simulink model "velocityform"  (R2024a)
settings: Solver=VariableStepAuto  StartTime=0.0  StopTime=10.0  RelTol=1e-3
values from neighbouring files (symbols this model uses):
  B_noise_real = [Bd ones(size(Bd,1),1)]    [scriptpoint7.m]
  D_noise_real = [Dd zeros(size(Dd,1),1)]    [scriptpoint7.m]
  N = 5    [project_script.m]    (also in scriptpoint7.m)
  NK = 0    [scriptpoint7.m]
  Qd = 1*eye(2)    [project_script.m]    (also in scriptpoint7.m = 1000*eye(2))
  Rd = 1*eye(2)    [project_script.m]    (also in scriptpoint7.m)
  RK = 1*eye(2)    [scriptpoint7.m]
  Ts = 1/8000    (= 0.000125)    [project_script.m]    (also in scriptpoint7.m)
  u_bar_d = Bd\ (eye(size(Ad))-Ad)*xref    [project_script.m]    (also in scriptpoint7.m)
  u_sat_max = [u1_max; u2_max]    [project_script.m]    (also in scriptpoint7.m)
  u_sat_min = [u1_min; u2_min]    [project_script.m]    (also in scriptpoint7.m)
  x0 = [x0_1;x0_2]    [project_script.m]    (also in scriptpoint7.m)
  x0K = 1.5*x0    [scriptpoint7.m]
  x_sat_max = [x1_max; x2_max]    [project_script.m]    (also in scriptpoint7.m)
  x_sat_min = [x1_min; x2_min]    [project_script.m]    (also in scriptpoint7.m)
  xref = [6.9; 8.9]    [project_script.m]    (also in scriptpoint7.m)
undefined symbols (not defined in the file or in its folder): Ad, Ad_real, Bd, Bd_real, Cd, Cd_real, Dd, Dd_real, Discrete, mympc, myvelocitympc, Sd, Time
libraries: simulink x4, ctrlSharedLib x2
settings Model: Creator=Utente  LastModifiedBy=Utente

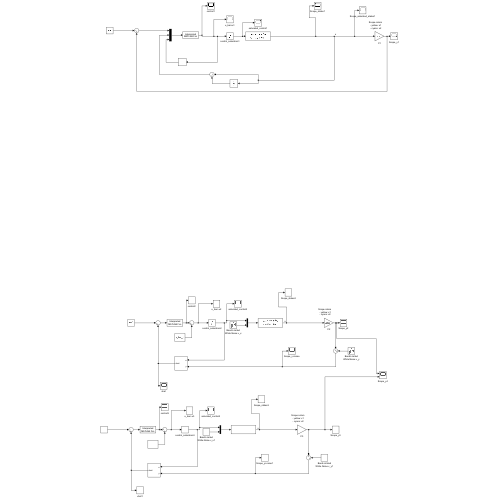
[thumbnail: Simulink's stored preview of the top-level diagram]
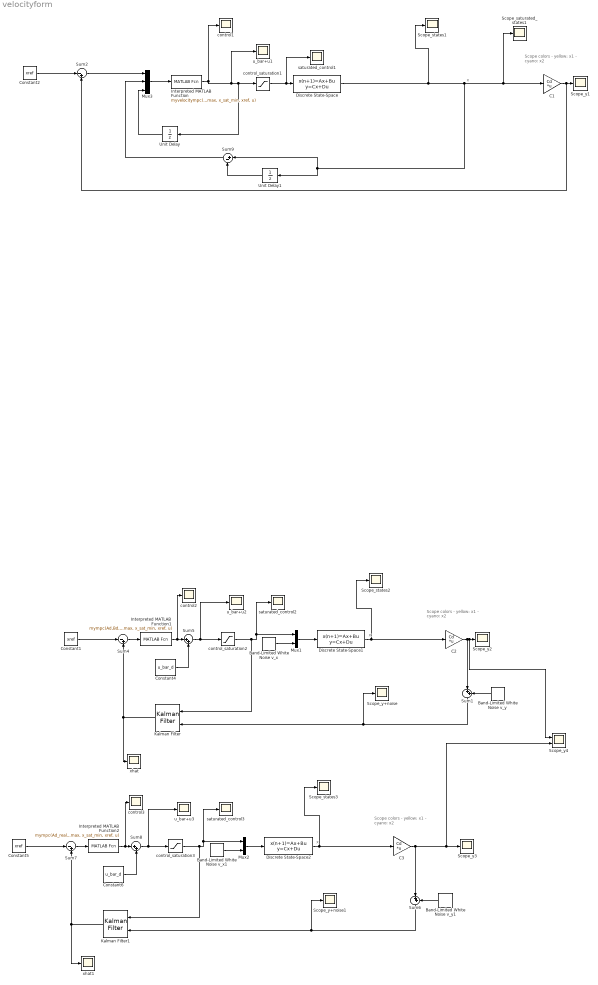
== system velocityform ==
  note: x
  note: Scope colors
      | - yellow: x1
      | - cyano: x2
  note: Scope colors
      | - yellow: x1
      | - cyano: x2
  note: x
  note: Scope colors
      | - yellow: x1
      | - cyano: x2
  note: x
  Band-Limited White Noise v_x : simulink/Sources/Band-Limited White Noise  Cov=power_vx  Ts=Ts  seed=[123]
  Band-Limited White Noise v_x1 : simulink/Sources/Band-Limited White Noise  Cov=power_vx  Ts=Ts  seed=[123]
  Band-Limited White Noise v_y : simulink/Sources/Band-Limited White Noise  Cov=power_vy  Ts=Ts  seed=[456]
  Band-Limited White Noise v_y1 : simulink/Sources/Band-Limited White Noise  Cov=power_vy  Ts=Ts  seed=[456]
  C1 : Gain  Gain=Cd  Multiplication=Matrix(K*u)
  C2 : Gain  Gain=Cd  Multiplication=Matrix(K*u)
  C3 : Gain  Gain=Cd  Multiplication=Matrix(K*u)
  Constant1 : Constant  Value=xref  SampleTime=Ts
  Constant2 : Constant  Value=xref  SampleTime=Ts
  Constant4 : Constant  Value=u_bar_d  SampleTime=Ts
  Constant5 : Constant  Value=xref  SampleTime=Ts
  Constant6 : Constant  Value=u_bar_d  SampleTime=Ts
  Discrete State-Space : DiscreteStateSpace  A=Ad  B=Bd  C=Cd  D=Dd  InitialCondition=x0  SampleTime=Ts
  Discrete State-Space1 : DiscreteStateSpace  A=Ad_real  B=B_noise_real  C=Cd_real  D=D_noise_real  InitialCondition=x0  SampleTime=Ts
  Discrete State-Space2 : DiscreteStateSpace  A=Ad_real  B=B_noise_real  C=Cd_real  D=D_noise_real  InitialCondition=x0  SampleTime=Ts
  Interpreted MATLAB Function : MATLABFcn  MATLABFcn=myvelocitympc(Ad,Bd,Cd,Qd,Rd,Sd,N,u_sat_min,u_sat_max,u_bar_d, x_sat_max, x_sat_min, xref, u)
  Interpreted MATLAB Function1 : MATLABFcn  MATLABFcn=mympc(Ad,Bd,Qd,Rd,Sd,N,u_sat_min,u_sat_max,u_bar_d, x_sat_max, x_sat_min, xref, u)
  Interpreted MATLAB Function2 : MATLABFcn  MATLABFcn=mympc(Ad_real,Bd_real,Qd,Rd,Sd,N,u_sat_min,u_sat_max,u_bar_d, x_sat_max, x_sat_min, xref, u)
  Kalman Filter : ctrlSharedLib/Kalman Filter  TimeDomain=Discrete-Time  UseCurrentEstimator=on  ModelSource=Individual A, B, C, D matrices  ModelSourceVariable=ss(0.95,1,1,0,1)  A=Ad  B=Bd  C=Cd  D=Dd  NumberOfStates=1  NumberOfInputs=1  NumberOfOutputs=1  InitialEstimateSource=Dialog  X0=x0K  P0=10  UseK=off  UseGH=off  NumberOfProcessNoiseInputs=1  G=1  TimeInvariantG=on  H=0  TimeInvariantH=on  Q=QK  TimeInvariantQ=on  R=RK  TimeInvariantR=on  N=NK  TimeInvariantN=on  AddInputPort=on  AddEnablePort=off  OutputEstimatedY=off  OutputP=off  Ts=-1
  Kalman Filter1 : ctrlSharedLib/Kalman Filter  TimeDomain=Discrete-Time  UseCurrentEstimator=on  ModelSource=Individual A, B, C, D matrices  ModelSourceVariable=ss(0.95,1,1,0,1)  A=Ad_real  B=Bd_real  C=Cd_real  D=Dd_real  NumberOfStates=1  NumberOfInputs=1  NumberOfOutputs=1  InitialEstimateSource=Dialog  X0=x0K  P0=10  UseK=off  UseGH=off  NumberOfProcessNoiseInputs=1  G=1  TimeInvariantG=on  H=0  TimeInvariantH=on  Q=QK  TimeInvariantQ=on  R=RK  TimeInvariantR=on  N=NK  TimeInvariantN=on  AddInputPort=on  AddEnablePort=off  OutputEstimatedY=off  OutputP=off  Ts=-1
  Mux1 : Mux  Inputs=2
  Mux2 : Mux  Inputs=2
  Mux3 : Mux  Inputs=3
  Scope_saturated_states1 : Scope
  Scope_states1 : Scope
  Scope_states2 : Scope
  Scope_states3 : Scope
  Scope_y+noise : Scope
  Scope_y+noise1 : Scope
  Scope_y1 : Scope
  Scope_y2 : Scope
  Scope_y3 : Scope
  Scope_y4 : Scope  NumInputPorts=2
  Sum{1,5..6,8} (4 alike) : Sum  Inputs=|++
  Sum2 : Sum  Inputs=|-+
  Sum4 : Sum  Inputs=|-+
  Sum7 : Sum  Inputs=|-+
  Sum9 : Sum  Inputs=|+-
  Unit Delay : UnitDelay  SampleTime=-1  HasFrameUpgradeWarning=on
  Unit Delay1 : UnitDelay  SampleTime=-1  HasFrameUpgradeWarning=on
  control1 : Scope
  control2 : Scope
  control3 : Scope
  control_saturation1 : Saturate  UpperLimit=u_sat_max  LowerLimit=u_sat_min
  control_saturation2 : Saturate  UpperLimit=u_sat_max  LowerLimit=u_sat_min
  control_saturation3 : Saturate  UpperLimit=u_sat_max  LowerLimit=u_sat_min
  saturated_control1 : Scope
  saturated_control2 : Scope
  saturated_control3 : Scope
  u_bar+u1 : Scope
  u_bar+u2 : Scope
  u_bar+u3 : Scope
  xhat : Scope
  xhat1 : Scope
  wires:
  Discrete State-Space/1 -> C1/1, Scope_saturated_states1/1, Sum9/1, Unit Delay1/1, Scope_states1/1
  C1/1 -> Sum2/2, Scope_y1/1
  Interpreted MATLAB Function/1 -> Unit Delay/1, control_saturation1/1, u_bar+u1/1, control1/1
  Constant2/1 -> Sum2/1
  control_saturation1/1 -> saturated_control1/1, Discrete State-Space/1
  Mux1/1 -> Discrete State-Space1/1
  Band-Limited White Noise v_x/1 -> Mux1/2
  Discrete State-Space1/1 -> C2/1, Scope_states2/1
  Sum5/1 -> control_saturation2/1, u_bar+u2/1
  Constant4/1 -> Sum5/2
  Band-Limited White Noise v_y/1 -> Sum1/2
  Kalman Filter/1 -> xhat/1, Sum4/2
  Interpreted MATLAB Function1/1 -> control2/1, Sum5/1
  Sum1/1 -> Kalman Filter/2, Scope_y+noise/1
  Constant1/1 -> Sum4/1
  Sum4/1 -> Interpreted MATLAB Function1/1
  control_saturation2/1 -> Kalman Filter/1, Mux1/1, saturated_control2/1
  C2/1 -> Scope_y4/1, Scope_y2/1, Sum1/1
  control_saturation3/1 -> Kalman Filter1/1, Mux2/1, saturated_control3/1
  C3/1 -> Scope_y4/2, Scope_y3/1, Sum6/1
  Interpreted MATLAB Function2/1 -> control3/1, Sum8/1
  Kalman Filter1/1 -> xhat1/1, Sum7/2
  Constant6/1 -> Sum8/2
  Sum7/1 -> Interpreted MATLAB Function2/1
  Constant5/1 -> Sum7/1
  Band-Limited White Noise v_y1/1 -> Sum6/2
  Sum8/1 -> control_saturation3/1, u_bar+u3/1
  Band-Limited White Noise v_x1/1 -> Mux2/2
  Mux2/1 -> Discrete State-Space2/1
  Sum6/1 -> Kalman Filter1/2, Scope_y+noise1/1
  Discrete State-Space2/1 -> C3/1, Scope_states3/1
  Mux3/1 -> Interpreted MATLAB Function/1
  Unit Delay1/1 -> Sum9/2
  Sum9/1 -> Mux3/2
  Sum2/1 -> Mux3/1
  Unit Delay/1 -> Mux3/3
